simulink model "filterbankOctaveProper"  (R2018a)
settings: Solver=FixedStepDiscrete  StartTime=0.0  StopTime=0.01  RelTol=1e-3
values from neighbouring files (symbols this model uses):
  gainConsts = 10.^(requiredGainDB/10)    [main.m]
  T = table(Band, fm, Lowerfreq, Upperfreq, Fstop2, Fstop1)    [filterbankProto.m]    (also in main.m = 2.26757369615e-05)
libraries: audiofilters x32, dspsrcs4 x2, dspfdesign x2, dspxfrm3 x1, dsparch4 x1, dspspect3 x1, dspsigops x1, dspmisc x1, dspmtrx3 x1, dspobslib x1
settings Model: Creator=Kavi  LastModifiedBy=kavilannair
settings SolverCC: AutoInsertRateTranBlk=on
settings DataIOCC: LimitDataPoints=on  SaveOutput=off  SignalLogging=off  SaveTime=off
settings OptimizationCC: LifeSpan=inf  SimCompilerOptimization=on
settings DebuggingCC: AlgebraicLoopMsg=error  SingleTaskRateTransMsg=error  AllowSymbolicDim=off  SFUnexpectedBacktrackingDiag=warning  SFNoUnconditionalDefaultTransitionDiag=warning  SFExecutionAtInitializationDiag=none
settings CodeAppCC: StateflowObjectComments=on
settings GRTTargetCC: TargetLangStandard=C89/C90 (ANSI)  GeneratePreprocessorConditionals=Disable all
settings ConfigComp: CovMetricSettings=dw  CovHtmlReporting=on  CovSaveCumulativeToWorkspaceVar=on  CovSaveSingleToWorkspaceVar=on  CovExternalEMLEnable=off  CovSFcnEnable=off

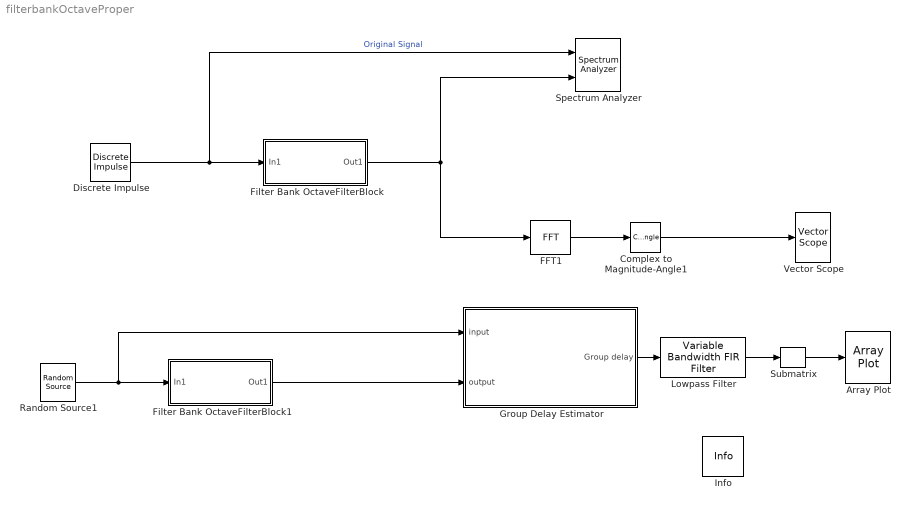
== system filterbankOctaveProper ==
  Array Plot : ArrayPlot
  Complex to Magnitude-Angle1 : ComplexToMagnitudeAngle  Output=Magnitude
  Discrete Impulse : dspsrcs4/Discrete  Impulse  Delay=0  SampleTime=T  FrameSample=512  OutputFrames=off  dataType=double  isSigned=on  wordLen=16  udDataType=sfix(16)  fracBitsMode=Best precision  numFracBits=15  OutDataTypeStr=double  LastOutDataTypeStr=double
  FFT1 : dspxfrm3/FFT  FFTImplementation=Auto  CompMethod=Table lookup  TableOpt=NEW  TableOptActive=Speed  BitRevOrder=off  Normalize=off  InheritFFTLength=on  FFTLength=64  WrapInput=on  roundingMode=Floor  overflowMode=off  firstCoeffDataTypeStr=Inherit: Same word length as input  firstCoeffLastDataTypeStr=Inherit: Same word length as input  outputMin=[]  outputMax=[]
  Filter Bank OctaveFilterBlock : Subsystem
  Filter Bank OctaveFilterBlock1 : Subsystem
  Group Delay Estimator : Subsystem
  Info : dspmisc/Info  SystemSampleTime=-1
      settings: SourceProductName=DSP System Toolbox  SourceProductBaseCode=DS
  Lowpass Filter : dspfdesign/Variable Bandwidth FIR Filter  FilterOrder=30  FilterType=Lowpass  CutoffFrequencyPort=off  CutoffFrequency=fc  CenterFrequencyPort=off  CenterFrequency=1e4  BandwidthPort=off  Bandwidth=2e3  Window=Hann  KaiserWindowParameter=.5  SidelobeAttenuation=60  InheritSampleRate=off  SampleRate=44100  SimulateUsing=Interpreted execution  mask(dsp.simulink.VariableBandwidthFIRFilter){fc=1323.094}
      mask prompts: fc "Cutoff frequency (Hz)"
      mask help: Masked version of dspfdesign/Variable Bandwidth FIR Filter block
      settings: SourceProductName=DSP System Toolbox  SourceProductBaseCode=DS
      mask Display:
      | % This is a new mask on top of the base mask.
      | % Use "View base mask" link below to see the base mask.
      | fprintf('Lowpass filter')
  Random Source1 : dspsrcs4/Random Source  SrcType=Gaussian  NormMethod=Ziggurat  CltLength=12  MinVal=0  MaxVal=1  MeanVal=0  VarVal=1  RepMode=Repeatable  rawSeed=1  IsInherit=off  SampMode=Discrete  SampTime=1/44100  SampFrame=512  DataType=Double  OutComplex=Real  OutputFrames=off
  Spectrum Analyzer : SpectrumAnalyzer  NumInputPorts=2
  Submatrix : dspmtrx3/Submatrix  RowSpan=Range of rows  RowStartMode=Index  RowStartIndex=31  RowEndMode=Last  RowEndIndex=1  ColSpan=All columns  ColStartMode=First  ColStartIndex=1  ColEndMode=Last  ColEndIndex=1
  Vector Scope : dspobslib/Vector Scope  ScopeProperties=off  Domain=Frequency  HorizSpan=1  DisplayProperties=off  AxisGrid=on  Memory=off  FrameNumber=on  AxisLegend=off  AxisZoom=off  OpenScopeAtSimStart=on  OpenScopeImmediately=off  FigPos=[412 353 1118 420]  AxisProperties=on  XUnits=Hertz  XRange=[0...Fs/2]  InheritXIncr=on  XIncr=1  XLabel=Samples  XLimit=Auto  XMin=0  XMax=1  XStart=0  YUnits=dB  YLabel=|Magnitude (dB)|  LineProperties=off  LineMarkers=+  LineColors=[1 0 0]  XAxisParamsVer=6.9
      settings: SourceProductName=DSP System Toolbox  SourceProductBaseCode=DS  YMin=0.0723692553519949  YMax=69.3188381671759
  wires:
  Discrete Impulse/1 -> Spectrum Analyzer/1, Filter Bank OctaveFilterBlock/1(In1)  "Original Signal"
  Complex to Magnitude-Angle1/1 -> Vector Scope/1
  FFT1/1 -> Complex to Magnitude-Angle1/1
  Filter Bank OctaveFilterBlock/1(Out1) -> FFT1/1, Spectrum Analyzer/2
  Filter Bank OctaveFilterBlock1/1(Out1) -> Group Delay Estimator/2(output)
  Group Delay Estimator/1(Group delay) -> Lowpass Filter/1
  Submatrix/1 -> Array Plot/1
  Lowpass Filter/1 -> Submatrix/1
  Random Source1/1 -> Group Delay Estimator/1(input), Filter Bank OctaveFilterBlock1/1(In1)

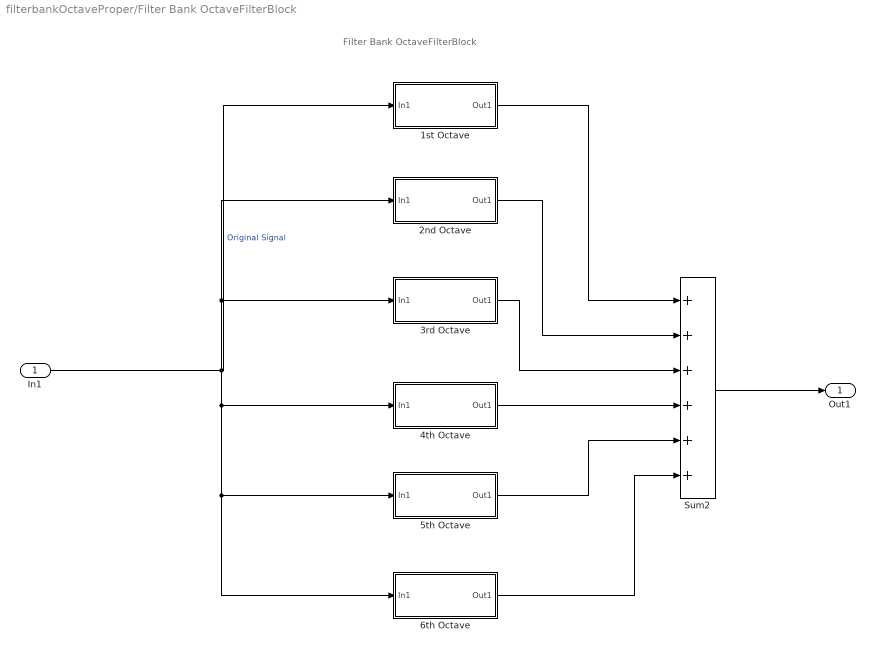
== system filterbankOctaveProper/Filter Bank OctaveFilterBlock ==
  note: Filter Bank OctaveFilterBlock
  In1 : Inport
  "1st Octave " : Subsystem
  2nd Octave : Subsystem
  "3rd Octave " : Subsystem
  4th Octave : Subsystem
  5th Octave : Subsystem
  6th Octave : Subsystem
  Sum2 : Sum  Inputs=++++++
  Out1 : Outport
  wires:
  Sum2/1 -> Out1/1
  "1st Octave "/1(Out1) -> Sum2/1
  2nd Octave/1(Out1) -> Sum2/2
  "3rd Octave "/1(Out1) -> Sum2/3
  4th Octave/1(Out1) -> Sum2/4
  5th Octave/1(Out1) -> Sum2/5
  6th Octave/1(Out1) -> Sum2/6
  In1/1 -> 4th Octave/1(In1), 5th Octave/1(In1), 6th Octave/1(In1), "3rd Octave "/1(In1), 2nd Octave/1(In1), "1st Octave "/1(In1)  "Original Signal"

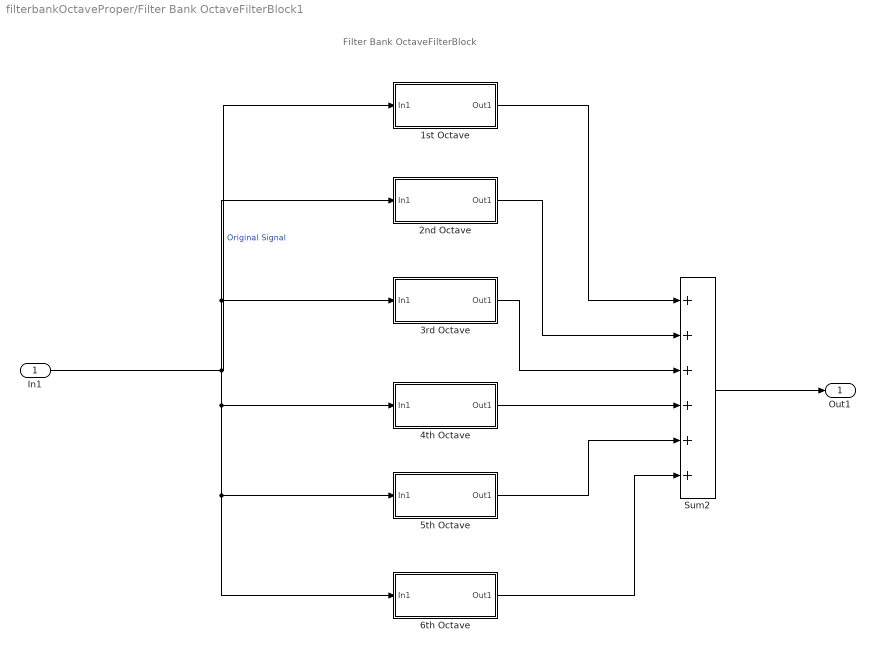
== system filterbankOctaveProper/Filter Bank OctaveFilterBlock1 ==
  note: Filter Bank OctaveFilterBlock
  In1 : Inport
  "1st Octave " : Subsystem
  2nd Octave : Subsystem
  "3rd Octave " : Subsystem
  4th Octave : Subsystem
  5th Octave : Subsystem
  6th Octave : Subsystem
  Sum2 : Sum  Inputs=++++++
  Out1 : Outport
  wires:
  Sum2/1 -> Out1/1
  "1st Octave "/1(Out1) -> Sum2/1
  2nd Octave/1(Out1) -> Sum2/2
  "3rd Octave "/1(Out1) -> Sum2/3
  4th Octave/1(Out1) -> Sum2/4
  5th Octave/1(Out1) -> Sum2/5
  6th Octave/1(Out1) -> Sum2/6
  In1/1 -> 4th Octave/1(In1), 5th Octave/1(In1), 6th Octave/1(In1), "3rd Octave "/1(In1), 2nd Octave/1(In1), "1st Octave "/1(In1)  "Original Signal"

== system filterbankOctaveProper/Group Delay Estimator ==
  input : Inport
  output : Inport  Port=2
  Differentiator Filter : dspfdesign/Differentiator Filter  DesignForMinimumOrder=off  FilterOrder=3  PassbandRipple=0.1  ScaleCoefficients=off  SimulateUsing=Interpreted execution  roundingMode=Floor  coeffsDataTypeStr=fixdt(1,16)
      settings: SourceProductName=DSP System Toolbox  SourceProductBaseCode=DS
  Discrete Transfer Function Estimator : dspspect3/Discrete Transfer Function Estimator  WindowLength=2056  Overlap=0  SpectralAverages=10  FFTLengthSource=Auto  FFTLength=2048  Window=Hann  SidelobeAttenuation=60  FrequencyRange=One-sided  OutputCoherence=off  SimulateUsing=Code generation
      settings: SourceProductName=DSP System Toolbox  SourceProductBaseCode=DS
  Gain1 : Gain  Gain=-22050/257
  Phase Extractor : dspsigops/Phase Extractor  TreatFramesIndependently=on  SimulateUsing=Code generation
      settings: SourceProductName=DSP System Toolbox  SourceProductBaseCode=DS
  Group delay : Outport
  wires:
  output/1 -> Discrete Transfer Function Estimator/2
  Differentiator Filter/1 -> Group delay/1
  input/1 -> Discrete Transfer Function Estimator/1
  Gain1/1 -> Differentiator Filter/1
  Phase Extractor/1 -> Gain1/1
  Discrete Transfer Function Estimator/1 -> Phase Extractor/1

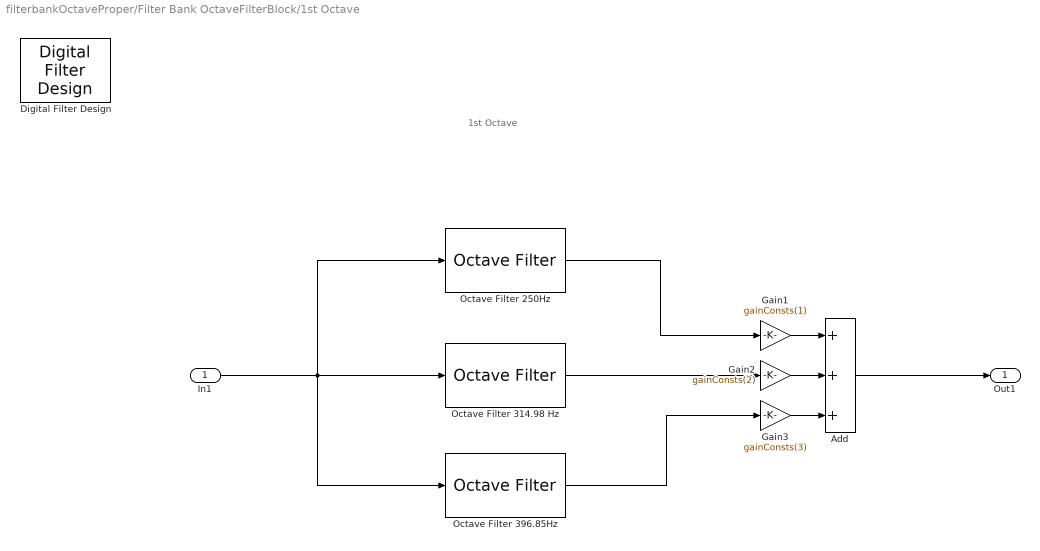
== system filterbankOctaveProper/Filter Bank OctaveFilterBlock/1st Octave  ==
  note: 1st Octave
  In1 : Inport
  Add : Sum  Inputs=+++
  Digital Filter Design : dsparch4/Digital Filter Design  mwdsp_browser_bugfix_var=off
  Gain1 : Gain  Gain=gainConsts(1)
  Gain2 : Gain  Gain=gainConsts(2)
  Gain3 : Gain  Gain=gainConsts(3)
  "Octave Filter 250Hz " : audiofilters/Octave Filter  FilterOrder=6  CenterFrequencyPort=off  CenterFrequency=250  Bandwidth=1 octave  BandsPerOctave=3  BandwidthType=1/3 octave  Oversample=off  InheritSampleRate=off  SampleRate=44100  SimulateUsing=Code generation  MaskClassType=Class 0
      settings: SourceProductName=Audio System Toolbox  SourceProductBaseCode=AU
  "Octave Filter 314.98 Hz " : audiofilters/Octave Filter  FilterOrder=6  CenterFrequencyPort=off  CenterFrequency=314.98  Bandwidth=1 octave  BandsPerOctave=3  BandwidthType=1/3 octave  Oversample=off  InheritSampleRate=off  SampleRate=44100  SimulateUsing=Code generation  MaskClassType=Class 0
      settings: SourceProductName=Audio System Toolbox  SourceProductBaseCode=AU
  "Octave Filter 396.85Hz " : audiofilters/Octave Filter  FilterOrder=6  CenterFrequencyPort=off  CenterFrequency=396.85  Bandwidth=1 octave  BandsPerOctave=3  BandwidthType=1/3 octave  Oversample=off  InheritSampleRate=off  SampleRate=44100  SimulateUsing=Code generation  MaskClassType=Class 0
      settings: SourceProductName=Audio System Toolbox  SourceProductBaseCode=AU
  Out1 : Outport
  wires:
  In1/1 -> "Octave Filter 250Hz "/1, "Octave Filter 314.98 Hz "/1, "Octave Filter 396.85Hz "/1
  "Octave Filter 314.98 Hz "/1 -> Gain2/1
  "Octave Filter 250Hz "/1 -> Gain1/1
  "Octave Filter 396.85Hz "/1 -> Gain3/1
  Add/1 -> Out1/1
  Gain1/1 -> Add/1
  Gain2/1 -> Add/2
  Gain3/1 -> Add/3

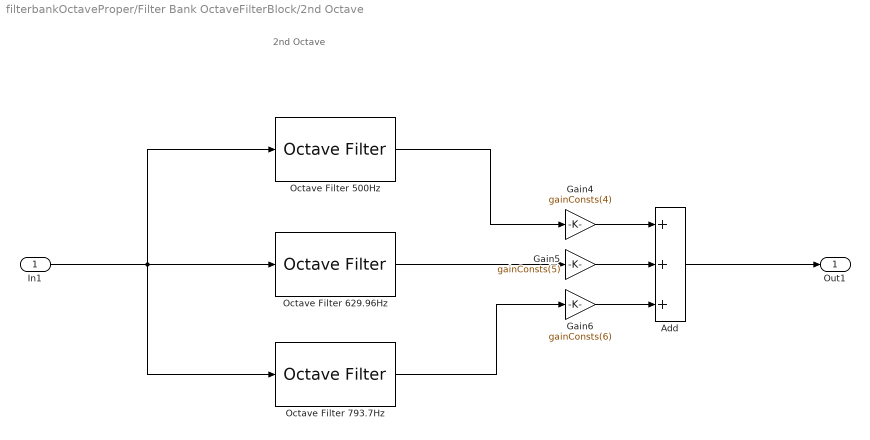
== system filterbankOctaveProper/Filter Bank OctaveFilterBlock/2nd Octave ==
  note: 2nd Octave
  In1 : Inport
  Add : Sum  Inputs=+++
  Gain4 : Gain  Gain=gainConsts(4)
  Gain5 : Gain  Gain=gainConsts(5)
  Gain6 : Gain  Gain=gainConsts(6)
  "Octave Filter 500Hz " : audiofilters/Octave Filter  FilterOrder=6  CenterFrequencyPort=off  CenterFrequency=500  Bandwidth=1 octave  BandsPerOctave=3  BandwidthType=1/3 octave  Oversample=off  InheritSampleRate=off  SampleRate=44100  SimulateUsing=Code generation  MaskClassType=Class 0
      settings: SourceProductName=Audio System Toolbox  SourceProductBaseCode=AU
  "Octave Filter 629.96Hz " : audiofilters/Octave Filter  FilterOrder=6  CenterFrequencyPort=off  CenterFrequency=629.96  Bandwidth=1 octave  BandsPerOctave=3  BandwidthType=1/3 octave  Oversample=off  InheritSampleRate=off  SampleRate=44100  SimulateUsing=Code generation  MaskClassType=Class 0
      settings: SourceProductName=Audio System Toolbox  SourceProductBaseCode=AU
  "Octave Filter 793.7Hz " : audiofilters/Octave Filter  FilterOrder=6  CenterFrequencyPort=off  CenterFrequency=793.7  Bandwidth=1 octave  BandsPerOctave=3  BandwidthType=1/3 octave  Oversample=off  InheritSampleRate=off  SampleRate=44100  SimulateUsing=Code generation  MaskClassType=Class 0
      settings: SourceProductName=Audio System Toolbox  SourceProductBaseCode=AU
  Out1 : Outport
  wires:
  In1/1 -> "Octave Filter 500Hz "/1, "Octave Filter 629.96Hz "/1, "Octave Filter 793.7Hz "/1
  "Octave Filter 629.96Hz "/1 -> Gain5/1
  "Octave Filter 500Hz "/1 -> Gain4/1
  "Octave Filter 793.7Hz "/1 -> Gain6/1
  Add/1 -> Out1/1
  Gain4/1 -> Add/1
  Gain5/1 -> Add/2
  Gain6/1 -> Add/3

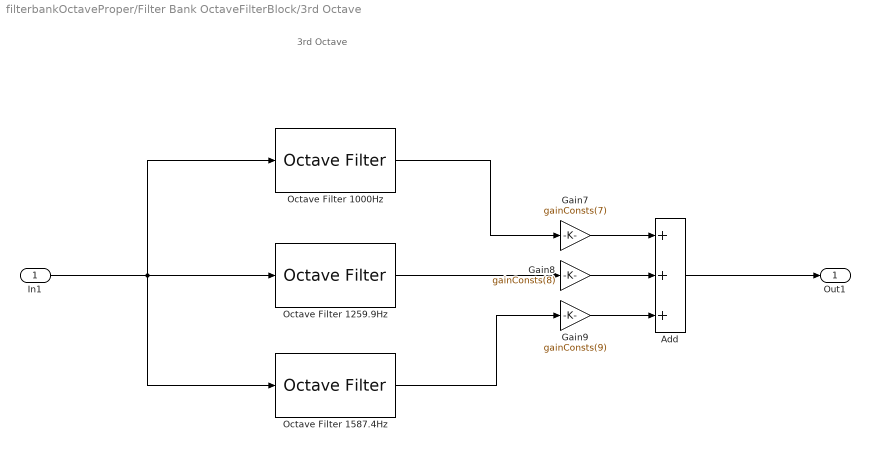
== system filterbankOctaveProper/Filter Bank OctaveFilterBlock/3rd Octave  ==
  note: 3rd Octave
  In1 : Inport
  Add : Sum  Inputs=+++
  Gain7 : Gain  Gain=gainConsts(7)
  Gain8 : Gain  Gain=gainConsts(8)
  Gain9 : Gain  Gain=gainConsts(9)
  "Octave Filter 1000Hz " : audiofilters/Octave Filter  FilterOrder=6  CenterFrequencyPort=off  CenterFrequency=1000  Bandwidth=1 octave  BandsPerOctave=3  BandwidthType=1/3 octave  Oversample=off  InheritSampleRate=off  SampleRate=44100  SimulateUsing=Code generation  MaskClassType=Class 0
      settings: SourceProductName=Audio System Toolbox  SourceProductBaseCode=AU
  "Octave Filter 1259.9Hz " : audiofilters/Octave Filter  FilterOrder=6  CenterFrequencyPort=off  CenterFrequency=314.98  Bandwidth=1 octave  BandsPerOctave=3  BandwidthType=1/3 octave  Oversample=off  InheritSampleRate=off  SampleRate=44100  SimulateUsing=Code generation  MaskClassType=Class 0
      settings: SourceProductName=Audio System Toolbox  SourceProductBaseCode=AU
  "Octave Filter 1587.4Hz " : audiofilters/Octave Filter  FilterOrder=6  CenterFrequencyPort=off  CenterFrequency=1587.4  Bandwidth=1 octave  BandsPerOctave=3  BandwidthType=1/3 octave  Oversample=off  InheritSampleRate=off  SampleRate=44100  SimulateUsing=Code generation  MaskClassType=Class 0
      settings: SourceProductName=Audio System Toolbox  SourceProductBaseCode=AU
  Out1 : Outport
  wires:
  In1/1 -> "Octave Filter 1000Hz "/1, "Octave Filter 1259.9Hz "/1, "Octave Filter 1587.4Hz "/1
  "Octave Filter 1259.9Hz "/1 -> Gain8/1
  "Octave Filter 1000Hz "/1 -> Gain7/1
  "Octave Filter 1587.4Hz "/1 -> Gain9/1
  Add/1 -> Out1/1
  Gain7/1 -> Add/1
  Gain8/1 -> Add/2
  Gain9/1 -> Add/3

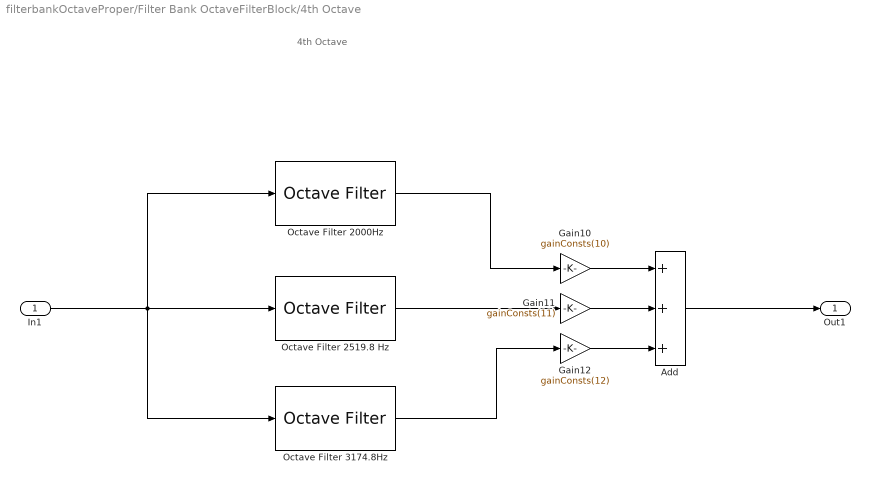
== system filterbankOctaveProper/Filter Bank OctaveFilterBlock/4th Octave ==
  note: 4th Octave
  In1 : Inport
  Add : Sum  Inputs=+++
  Gain10 : Gain  Gain=gainConsts(10)
  Gain11 : Gain  Gain=gainConsts(11)
  Gain12 : Gain  Gain=gainConsts(12)
  "Octave Filter 2000Hz " : audiofilters/Octave Filter  FilterOrder=6  CenterFrequencyPort=off  CenterFrequency=2000  Bandwidth=1 octave  BandsPerOctave=3  BandwidthType=1/3 octave  Oversample=off  InheritSampleRate=off  SampleRate=44100  SimulateUsing=Code generation  MaskClassType=Class 0
      settings: SourceProductName=Audio System Toolbox  SourceProductBaseCode=AU
  "Octave Filter 2519.8 Hz " : audiofilters/Octave Filter  FilterOrder=6  CenterFrequencyPort=off  CenterFrequency=2519.8  Bandwidth=1 octave  BandsPerOctave=3  BandwidthType=1/3 octave  Oversample=off  InheritSampleRate=off  SampleRate=44100  SimulateUsing=Code generation  MaskClassType=Class 0
      settings: SourceProductName=Audio System Toolbox  SourceProductBaseCode=AU
  "Octave Filter 3174.8Hz " : audiofilters/Octave Filter  FilterOrder=6  CenterFrequencyPort=off  CenterFrequency=3174.8  Bandwidth=1 octave  BandsPerOctave=3  BandwidthType=1/3 octave  Oversample=off  InheritSampleRate=off  SampleRate=44100  SimulateUsing=Code generation  MaskClassType=Class 0
      settings: SourceProductName=Audio System Toolbox  SourceProductBaseCode=AU
  Out1 : Outport
  wires:
  In1/1 -> "Octave Filter 2000Hz "/1, "Octave Filter 2519.8 Hz "/1, "Octave Filter 3174.8Hz "/1
  "Octave Filter 2519.8 Hz "/1 -> Gain11/1
  "Octave Filter 2000Hz "/1 -> Gain10/1
  "Octave Filter 3174.8Hz "/1 -> Gain12/1
  Add/1 -> Out1/1
  Gain10/1 -> Add/1
  Gain11/1 -> Add/2
  Gain12/1 -> Add/3

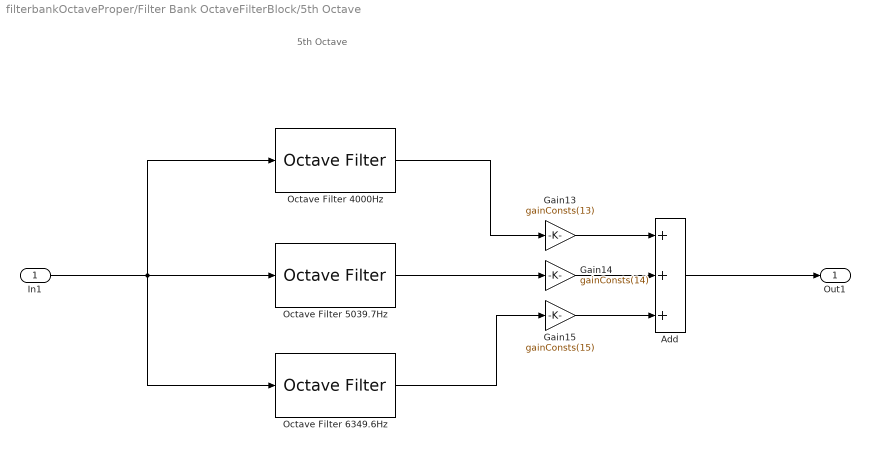
== system filterbankOctaveProper/Filter Bank OctaveFilterBlock/5th Octave ==
  note: 5th Octave
  In1 : Inport
  Add : Sum  Inputs=+++
  "Gain13 " : Gain  Gain=gainConsts(13)
  Gain14 : Gain  Gain=gainConsts(14)
  Gain15 : Gain  Gain=gainConsts(15)
  "Octave Filter 4000Hz " : audiofilters/Octave Filter  FilterOrder=6  CenterFrequencyPort=off  CenterFrequency=4000  Bandwidth=1 octave  BandsPerOctave=3  BandwidthType=1/3 octave  Oversample=off  InheritSampleRate=off  SampleRate=44100  SimulateUsing=Code generation  MaskClassType=Class 0
      settings: SourceProductName=Audio System Toolbox  SourceProductBaseCode=AU
  "Octave Filter 5039.7Hz " : audiofilters/Octave Filter  FilterOrder=6  CenterFrequencyPort=off  CenterFrequency=5039.7  Bandwidth=1 octave  BandsPerOctave=3  BandwidthType=1/3 octave  Oversample=off  InheritSampleRate=off  SampleRate=44100  SimulateUsing=Code generation  MaskClassType=Class 0
      settings: SourceProductName=Audio System Toolbox  SourceProductBaseCode=AU
  "Octave Filter 6349.6Hz " : audiofilters/Octave Filter  FilterOrder=6  CenterFrequencyPort=off  CenterFrequency=6349.6  Bandwidth=1 octave  BandsPerOctave=3  BandwidthType=1/3 octave  Oversample=off  InheritSampleRate=off  SampleRate=44100  SimulateUsing=Code generation  MaskClassType=Class 0
      settings: SourceProductName=Audio System Toolbox  SourceProductBaseCode=AU
  Out1 : Outport
  wires:
  In1/1 -> "Octave Filter 4000Hz "/1, "Octave Filter 5039.7Hz "/1, "Octave Filter 6349.6Hz "/1
  "Octave Filter 5039.7Hz "/1 -> Gain14/1
  "Octave Filter 4000Hz "/1 -> "Gain13 "/1
  "Octave Filter 6349.6Hz "/1 -> Gain15/1
  Add/1 -> Out1/1
  "Gain13 "/1 -> Add/1
  Gain14/1 -> Add/2
  Gain15/1 -> Add/3

== system filterbankOctaveProper/Filter Bank OctaveFilterBlock/6th Octave ==
  note: 6th Octave
  In1 : Inport
  Gain16 : Gain  Gain=gainConsts(16)
  "Octave Filter 8000Hz " : audiofilters/Octave Filter  FilterOrder=6  CenterFrequencyPort=off  CenterFrequency=8000  Bandwidth=1 octave  BandsPerOctave=3  BandwidthType=1/3 octave  Oversample=off  InheritSampleRate=off  SampleRate=44100  SimulateUsing=Code generation  MaskClassType=No mask
      settings: SourceProductName=Audio System Toolbox  SourceProductBaseCode=AU
  Out1 : Outport
  wires:
  In1/1 -> "Octave Filter 8000Hz "/1
  "Octave Filter 8000Hz "/1 -> Gain16/1
  Gain16/1 -> Out1/1

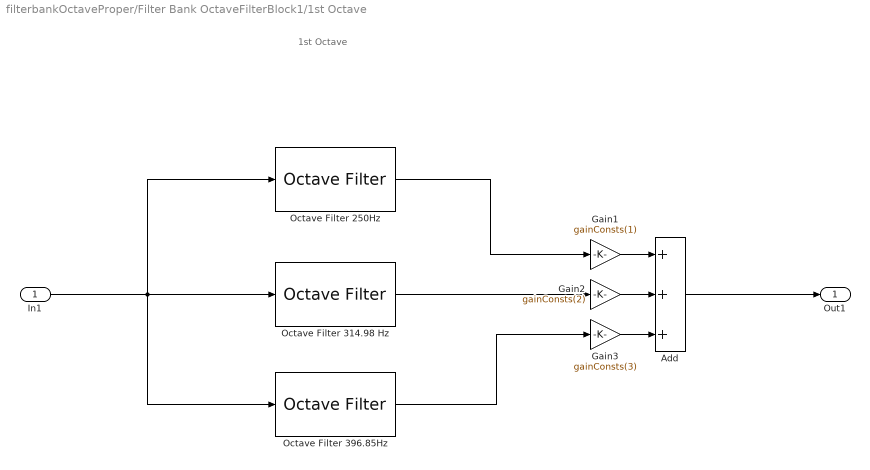
== system filterbankOctaveProper/Filter Bank OctaveFilterBlock1/1st Octave  ==
  note: 1st Octave
  In1 : Inport
  Add : Sum  Inputs=+++
  Gain1 : Gain  Gain=gainConsts(1)
  Gain2 : Gain  Gain=gainConsts(2)
  Gain3 : Gain  Gain=gainConsts(3)
  "Octave Filter 250Hz " : audiofilters/Octave Filter  FilterOrder=6  CenterFrequencyPort=off  CenterFrequency=250  Bandwidth=1 octave  BandsPerOctave=3  BandwidthType=1/3 octave  Oversample=off  InheritSampleRate=off  SampleRate=44100  SimulateUsing=Code generation  MaskClassType=Class 0
      settings: SourceProductName=Audio System Toolbox  SourceProductBaseCode=AU
  "Octave Filter 314.98 Hz " : audiofilters/Octave Filter  FilterOrder=6  CenterFrequencyPort=off  CenterFrequency=314.98  Bandwidth=1 octave  BandsPerOctave=3  BandwidthType=1/3 octave  Oversample=off  InheritSampleRate=off  SampleRate=44100  SimulateUsing=Code generation  MaskClassType=Class 0
      settings: SourceProductName=Audio System Toolbox  SourceProductBaseCode=AU
  "Octave Filter 396.85Hz " : audiofilters/Octave Filter  FilterOrder=6  CenterFrequencyPort=off  CenterFrequency=396.85  Bandwidth=1 octave  BandsPerOctave=3  BandwidthType=1/3 octave  Oversample=off  InheritSampleRate=off  SampleRate=44100  SimulateUsing=Code generation  MaskClassType=Class 0
      settings: SourceProductName=Audio System Toolbox  SourceProductBaseCode=AU
  Out1 : Outport
  wires:
  In1/1 -> "Octave Filter 250Hz "/1, "Octave Filter 314.98 Hz "/1, "Octave Filter 396.85Hz "/1
  "Octave Filter 314.98 Hz "/1 -> Gain2/1
  "Octave Filter 250Hz "/1 -> Gain1/1
  "Octave Filter 396.85Hz "/1 -> Gain3/1
  Add/1 -> Out1/1
  Gain1/1 -> Add/1
  Gain2/1 -> Add/2
  Gain3/1 -> Add/3

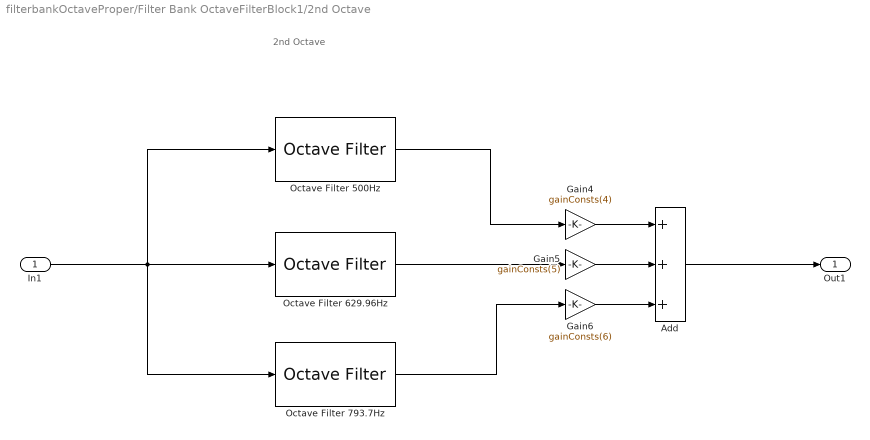
== system filterbankOctaveProper/Filter Bank OctaveFilterBlock1/2nd Octave ==
  note: 2nd Octave
  In1 : Inport
  Add : Sum  Inputs=+++
  Gain4 : Gain  Gain=gainConsts(4)
  Gain5 : Gain  Gain=gainConsts(5)
  Gain6 : Gain  Gain=gainConsts(6)
  "Octave Filter 500Hz " : audiofilters/Octave Filter  FilterOrder=6  CenterFrequencyPort=off  CenterFrequency=500  Bandwidth=1 octave  BandsPerOctave=3  BandwidthType=1/3 octave  Oversample=off  InheritSampleRate=off  SampleRate=44100  SimulateUsing=Code generation  MaskClassType=Class 0
      settings: SourceProductName=Audio System Toolbox  SourceProductBaseCode=AU
  "Octave Filter 629.96Hz " : audiofilters/Octave Filter  FilterOrder=6  CenterFrequencyPort=off  CenterFrequency=629.96  Bandwidth=1 octave  BandsPerOctave=3  BandwidthType=1/3 octave  Oversample=off  InheritSampleRate=off  SampleRate=44100  SimulateUsing=Code generation  MaskClassType=Class 0
      settings: SourceProductName=Audio System Toolbox  SourceProductBaseCode=AU
  "Octave Filter 793.7Hz " : audiofilters/Octave Filter  FilterOrder=6  CenterFrequencyPort=off  CenterFrequency=793.7  Bandwidth=1 octave  BandsPerOctave=3  BandwidthType=1/3 octave  Oversample=off  InheritSampleRate=off  SampleRate=44100  SimulateUsing=Code generation  MaskClassType=Class 0
      settings: SourceProductName=Audio System Toolbox  SourceProductBaseCode=AU
  Out1 : Outport
  wires:
  In1/1 -> "Octave Filter 500Hz "/1, "Octave Filter 629.96Hz "/1, "Octave Filter 793.7Hz "/1
  "Octave Filter 629.96Hz "/1 -> Gain5/1
  "Octave Filter 500Hz "/1 -> Gain4/1
  "Octave Filter 793.7Hz "/1 -> Gain6/1
  Add/1 -> Out1/1
  Gain4/1 -> Add/1
  Gain5/1 -> Add/2
  Gain6/1 -> Add/3

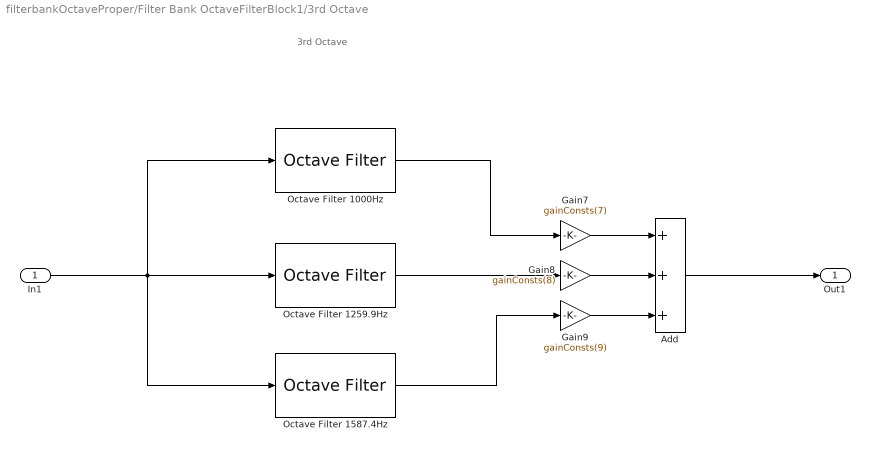
== system filterbankOctaveProper/Filter Bank OctaveFilterBlock1/3rd Octave  ==
  note: 3rd Octave
  In1 : Inport
  Add : Sum  Inputs=+++
  Gain7 : Gain  Gain=gainConsts(7)
  Gain8 : Gain  Gain=gainConsts(8)
  Gain9 : Gain  Gain=gainConsts(9)
  "Octave Filter 1000Hz " : audiofilters/Octave Filter  FilterOrder=6  CenterFrequencyPort=off  CenterFrequency=1000  Bandwidth=1 octave  BandsPerOctave=3  BandwidthType=1/3 octave  Oversample=off  InheritSampleRate=off  SampleRate=44100  SimulateUsing=Code generation  MaskClassType=Class 0
      settings: SourceProductName=Audio System Toolbox  SourceProductBaseCode=AU
  "Octave Filter 1259.9Hz " : audiofilters/Octave Filter  FilterOrder=6  CenterFrequencyPort=off  CenterFrequency=314.98  Bandwidth=1 octave  BandsPerOctave=3  BandwidthType=1/3 octave  Oversample=off  InheritSampleRate=off  SampleRate=44100  SimulateUsing=Code generation  MaskClassType=Class 0
      settings: SourceProductName=Audio System Toolbox  SourceProductBaseCode=AU
  "Octave Filter 1587.4Hz " : audiofilters/Octave Filter  FilterOrder=6  CenterFrequencyPort=off  CenterFrequency=1587.4  Bandwidth=1 octave  BandsPerOctave=3  BandwidthType=1/3 octave  Oversample=off  InheritSampleRate=off  SampleRate=44100  SimulateUsing=Code generation  MaskClassType=Class 0
      settings: SourceProductName=Audio System Toolbox  SourceProductBaseCode=AU
  Out1 : Outport
  wires:
  In1/1 -> "Octave Filter 1000Hz "/1, "Octave Filter 1259.9Hz "/1, "Octave Filter 1587.4Hz "/1
  "Octave Filter 1259.9Hz "/1 -> Gain8/1
  "Octave Filter 1000Hz "/1 -> Gain7/1
  "Octave Filter 1587.4Hz "/1 -> Gain9/1
  Add/1 -> Out1/1
  Gain7/1 -> Add/1
  Gain8/1 -> Add/2
  Gain9/1 -> Add/3

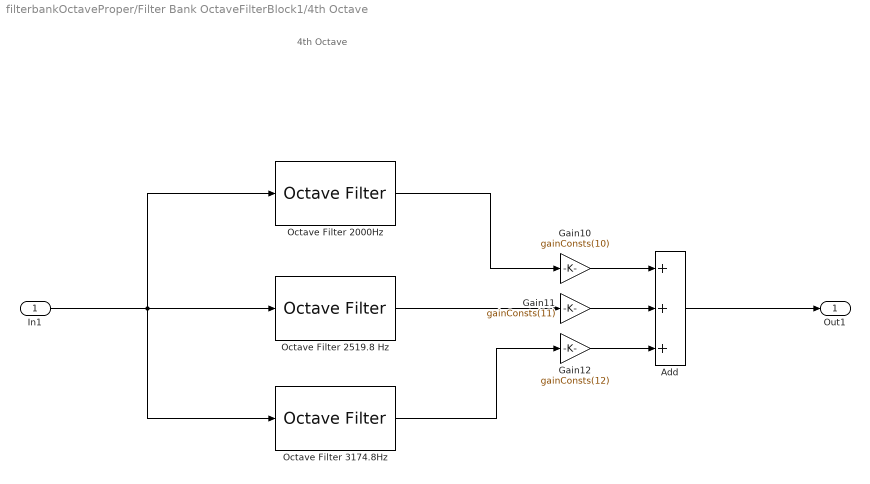
== system filterbankOctaveProper/Filter Bank OctaveFilterBlock1/4th Octave ==
  note: 4th Octave
  In1 : Inport
  Add : Sum  Inputs=+++
  Gain10 : Gain  Gain=gainConsts(10)
  Gain11 : Gain  Gain=gainConsts(11)
  Gain12 : Gain  Gain=gainConsts(12)
  "Octave Filter 2000Hz " : audiofilters/Octave Filter  FilterOrder=6  CenterFrequencyPort=off  CenterFrequency=2000  Bandwidth=1 octave  BandsPerOctave=3  BandwidthType=1/3 octave  Oversample=off  InheritSampleRate=off  SampleRate=44100  SimulateUsing=Code generation  MaskClassType=Class 0
      settings: SourceProductName=Audio System Toolbox  SourceProductBaseCode=AU
  "Octave Filter 2519.8 Hz " : audiofilters/Octave Filter  FilterOrder=6  CenterFrequencyPort=off  CenterFrequency=2519.8  Bandwidth=1 octave  BandsPerOctave=3  BandwidthType=1/3 octave  Oversample=off  InheritSampleRate=off  SampleRate=44100  SimulateUsing=Code generation  MaskClassType=Class 0
      settings: SourceProductName=Audio System Toolbox  SourceProductBaseCode=AU
  "Octave Filter 3174.8Hz " : audiofilters/Octave Filter  FilterOrder=6  CenterFrequencyPort=off  CenterFrequency=3174.8  Bandwidth=1 octave  BandsPerOctave=3  BandwidthType=1/3 octave  Oversample=off  InheritSampleRate=off  SampleRate=44100  SimulateUsing=Code generation  MaskClassType=Class 0
      settings: SourceProductName=Audio System Toolbox  SourceProductBaseCode=AU
  Out1 : Outport
  wires:
  In1/1 -> "Octave Filter 2000Hz "/1, "Octave Filter 2519.8 Hz "/1, "Octave Filter 3174.8Hz "/1
  "Octave Filter 2519.8 Hz "/1 -> Gain11/1
  "Octave Filter 2000Hz "/1 -> Gain10/1
  "Octave Filter 3174.8Hz "/1 -> Gain12/1
  Add/1 -> Out1/1
  Gain10/1 -> Add/1
  Gain11/1 -> Add/2
  Gain12/1 -> Add/3

== system filterbankOctaveProper/Filter Bank OctaveFilterBlock1/5th Octave ==
  note: 5th Octave
  In1 : Inport
  Add : Sum  Inputs=+++
  "Gain13 " : Gain  Gain=gainConsts(13)
  Gain14 : Gain  Gain=gainConsts(14)
  Gain15 : Gain  Gain=gainConsts(15)
  "Octave Filter 4000Hz " : audiofilters/Octave Filter  FilterOrder=6  CenterFrequencyPort=off  CenterFrequency=4000  Bandwidth=1 octave  BandsPerOctave=3  BandwidthType=1/3 octave  Oversample=off  InheritSampleRate=off  SampleRate=44100  SimulateUsing=Code generation  MaskClassType=Class 0
      settings: SourceProductName=Audio System Toolbox  SourceProductBaseCode=AU
  "Octave Filter 5039.7Hz " : audiofilters/Octave Filter  FilterOrder=6  CenterFrequencyPort=off  CenterFrequency=5039.7  Bandwidth=1 octave  BandsPerOctave=3  BandwidthType=1/3 octave  Oversample=off  InheritSampleRate=off  SampleRate=44100  SimulateUsing=Code generation  MaskClassType=Class 0
      settings: SourceProductName=Audio System Toolbox  SourceProductBaseCode=AU
  "Octave Filter 6349.6Hz " : audiofilters/Octave Filter  FilterOrder=6  CenterFrequencyPort=off  CenterFrequency=6349.6  Bandwidth=1 octave  BandsPerOctave=3  BandwidthType=1/3 octave  Oversample=off  InheritSampleRate=off  SampleRate=44100  SimulateUsing=Code generation  MaskClassType=Class 0
      settings: SourceProductName=Audio System Toolbox  SourceProductBaseCode=AU
  Out1 : Outport
  wires:
  In1/1 -> "Octave Filter 4000Hz "/1, "Octave Filter 5039.7Hz "/1, "Octave Filter 6349.6Hz "/1
  "Octave Filter 5039.7Hz "/1 -> Gain14/1
  "Octave Filter 4000Hz "/1 -> "Gain13 "/1
  "Octave Filter 6349.6Hz "/1 -> Gain15/1
  Add/1 -> Out1/1
  "Gain13 "/1 -> Add/1
  Gain14/1 -> Add/2
  Gain15/1 -> Add/3

== system filterbankOctaveProper/Filter Bank OctaveFilterBlock1/6th Octave ==
  note: 6th Octave
  In1 : Inport
  Gain16 : Gain  Gain=gainConsts(16)
  "Octave Filter 8000Hz " : audiofilters/Octave Filter  FilterOrder=6  CenterFrequencyPort=off  CenterFrequency=8000  Bandwidth=1 octave  BandsPerOctave=3  BandwidthType=1/3 octave  Oversample=off  InheritSampleRate=off  SampleRate=44100  SimulateUsing=Code generation  MaskClassType=No mask
      settings: SourceProductName=Audio System Toolbox  SourceProductBaseCode=AU
  Out1 : Outport
  wires:
  In1/1 -> "Octave Filter 8000Hz "/1
  "Octave Filter 8000Hz "/1 -> Gain16/1
  Gain16/1 -> Out1/1
